simulink model "ClampledRollPID"  (R2025b)
settings: Solver=VariableStepAuto  StartTime=0.0  StopTime=10  RelTol=1e-3
model workspace (MAT data in the model file):
  Dmass = 0.25
  Ix = 0.01
  Iy = 0.01
  Iz = 0.022
  Kd_h = 0
  Kd_r = 5
  Kd_y = 0
  Ki_h = 0
  Ki_r = 1
  Ki_y = 0
  Kp_h = 1
  Kp_r = 4
  Kp_y = 1
  d_m = 1
  d_pitch = 1
  d_roll = 1
  d_yaw = 1
libraries: simulink_extras x1
settings Model: Creator=mariea  LastModifiedBy=mariea
settings SolverCC: ZeroCrossAlgorithm=Adaptive
settings DebuggingCC: IgnoredZcDiagnostic=none

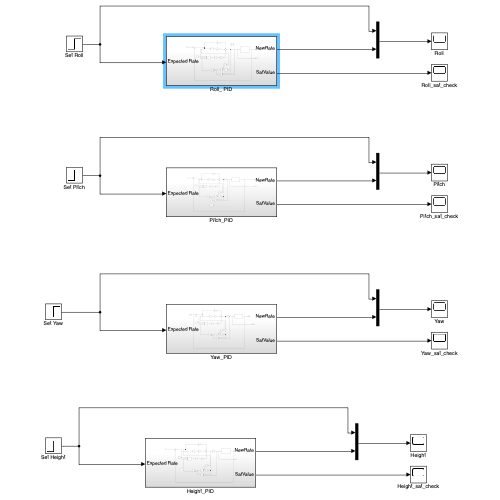
[thumbnail: Simulink's stored preview of the top-level diagram]
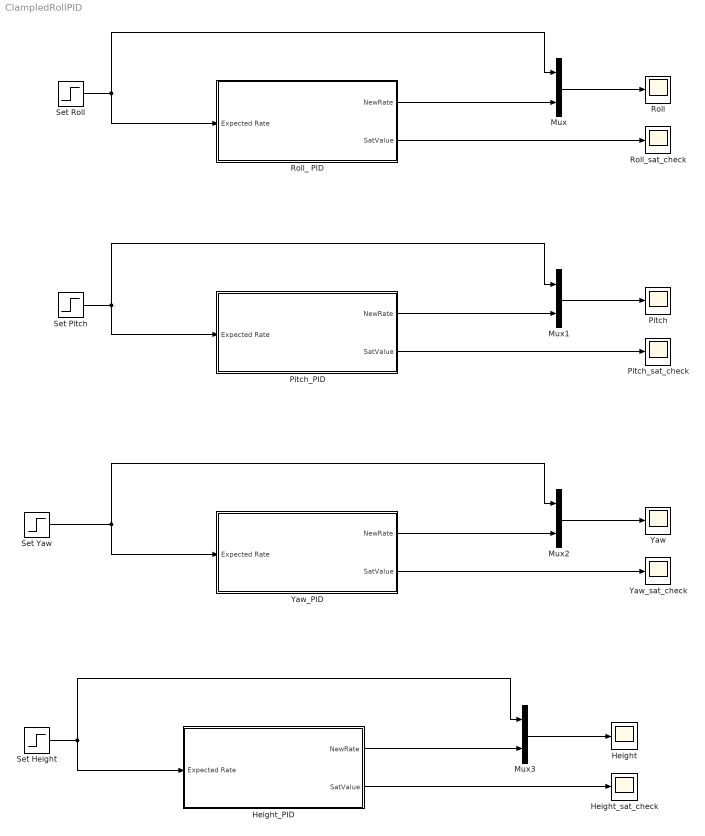
== system ClampledRollPID ==
  Height : Scope
      settings: ActiveDisplayYMinimum=-0.60536887029310371  ActiveDisplayYMaximum=10.192601111350347  DataLoggingVariableName=ScopeData6
  Height_PID : Subsystem
  Height_sat_check : Scope
      settings: ActiveDisplayYMinimum=2.8893405946008759  ActiveDisplayYMaximum=23.442208925875939  DataLoggingVariableName=ScopeData7
  Mux{,1..3} (4 alike) : Mux  Inputs=2
  Pitch : Scope
      settings: ActiveDisplayYMinimum=-0.60536887029310371  ActiveDisplayYMaximum=10.192601111350347  DataLoggingVariableName=ScopeData2
  Pitch_PID : Subsystem
  Pitch_sat_check : Scope
      settings: ActiveDisplayYMinimum=2.8893405946008759  ActiveDisplayYMaximum=23.442208925875939  DataLoggingVariableName=ScopeData3
  Roll : Scope
      settings: ActiveDisplayYMinimum=4.5448731516349712  ActiveDisplayYMaximum=5.1235702214097891
  Roll_ PID : Subsystem
  Roll_sat_check : Scope
      settings: ActiveDisplayYMinimum=-77.252153315942437  ActiveDisplayYMaximum=63.048289708603093
  Set Height : Step  After=3  SampleTime=0
  Set Pitch : Step  After=5  SampleTime=0
  Set Roll : Step  After=10  SampleTime=0
  Set Yaw : Step  After=7  SampleTime=0
  Yaw : Scope
      settings: ActiveDisplayYMinimum=-1.8749999999999996  ActiveDisplayYMaximum=16.875  DataLoggingVariableName=ScopeData4
  Yaw_PID : Subsystem
  Yaw_sat_check : Scope
      settings: ActiveDisplayYMinimum=2.8893405946008759  ActiveDisplayYMaximum=23.442208925875939  DataLoggingVariableName=ScopeData5
  wires:
  Set Roll/1 -> Roll_ PID/1(Expected Rate), Mux/1
  Mux/1 -> Roll/1
  Roll_ PID/1(NewRate) -> Mux/2
  Roll_ PID/2(SatValue) -> Roll_sat_check/1
  Set Pitch/1 -> Pitch_PID/1(Expected Rate), Mux1/1
  Pitch_PID/1(NewRate) -> Mux1/2
  Pitch_PID/2(SatValue) -> Pitch_sat_check/1
  Mux1/1 -> Pitch/1
  Mux2/1 -> Yaw/1
  Yaw_PID/1(NewRate) -> Mux2/2
  Set Yaw/1 -> Yaw_PID/1(Expected Rate), Mux2/1
  Yaw_PID/2(SatValue) -> Yaw_sat_check/1
  Mux3/1 -> Height/1
  Height_PID/1(NewRate) -> Mux3/2
  Set Height/1 -> Height_PID/1(Expected Rate), Mux3/1
  Height_PID/2(SatValue) -> Height_sat_check/1

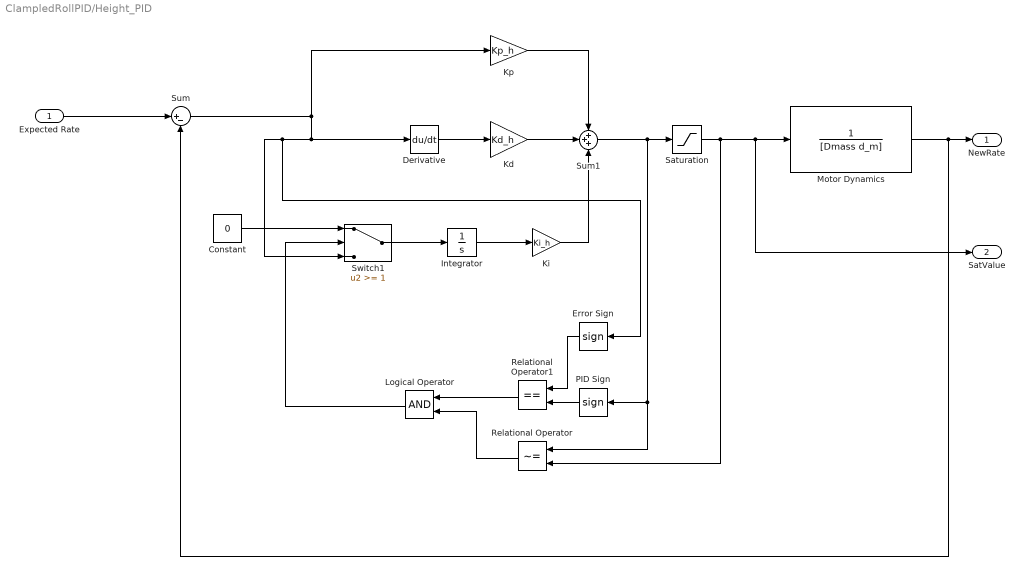
== system ClampledRollPID/Height_PID ==
  Expected Rate : Inport
  Constant : Constant  Value=0
  Derivative : Derivative
  Error Sign : Signum
  Integrator : Integrator
  Kd : Gain  Gain=Kd_h
  Ki : Gain  Gain=Ki_h
  Kp : Gain  Gain=Kp_h
  Logical Operator : Logic  AllPortsSameDT=off  OutDataTypeStr=boolean
  Motor Dynamics : TransferFcn  Denominator=[Dmass d_m]
  PID Sign : Signum
  Relational Operator : RelationalOperator  Operator=~=  OutDataTypeStr=boolean  RndMeth=Simplest  InputSameDT=off
  Relational Operator1 : RelationalOperator  Operator===  OutDataTypeStr=boolean  RndMeth=Simplest  InputSameDT=off
  Saturation : Saturate  UpperLimit=100  LowerLimit=0
  Sum : Sum  Inputs=|+-
  Sum1 : Sum  Inputs=+++
  Switch1 : Switch  Threshold=1  SaturateOnIntegerOverflow=off  InputSameDT=off
  NewRate : Outport
  SatValue : Outport  Port=2
  wires:
  Logical Operator/1 -> Switch1/2
  Kp/1 -> Sum1/1
  Error Sign/1 -> Relational Operator1/1
  Integrator/1 -> Ki/1
  Sum/1 -> Error Sign/1, Switch1/3, Derivative/1, Kp/1
  Switch1/1 -> Integrator/1
  Expected Rate/1 -> Sum/1
  Kd/1 -> Sum1/2
  Ki/1 -> Sum1/3
  Derivative/1 -> Kd/1
  Constant/1 -> Switch1/1
  Relational Operator1/1 -> Logical Operator/1
  Sum1/1 -> Saturation/1, PID Sign/1, Relational Operator/1
  PID Sign/1 -> Relational Operator1/2
  Relational Operator/1 -> Logical Operator/2
  Saturation/1 -> Relational Operator/2, SatValue/1, Motor Dynamics/1
  Motor Dynamics/1 -> Sum/2, NewRate/1

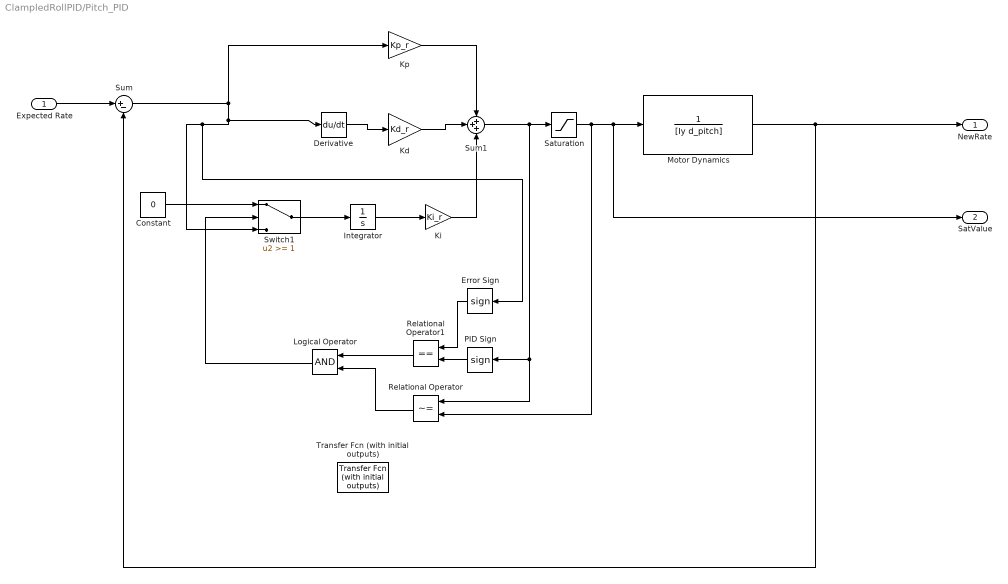
== system ClampledRollPID/Pitch_PID ==
  Expected Rate : Inport
  Constant : Constant  Value=0
  Derivative : Derivative
  Error Sign : Signum
  Integrator : Integrator
  Kd : Gain  Gain=Kd_r
  Ki : Gain  Gain=Ki_r
  Kp : Gain  Gain=Kp_r
  Logical Operator : Logic  AllPortsSameDT=off  OutDataTypeStr=boolean
  Motor Dynamics : TransferFcn  Denominator=[Iy d_pitch]
  PID Sign : Signum
  Relational Operator : RelationalOperator  Operator=~=  OutDataTypeStr=boolean  RndMeth=Simplest  InputSameDT=off
  Relational Operator1 : RelationalOperator  Operator===  OutDataTypeStr=boolean  RndMeth=Simplest  InputSameDT=off
  Saturation : Saturate  UpperLimit=96  LowerLimit=-96
  Sum : Sum  Inputs=|+-
  Sum1 : Sum  Inputs=+++
  Switch1 : Switch  Threshold=1  SaturateOnIntegerOverflow=off  InputSameDT=off
  Transfer Fcn (with initial outputs) : simulink_extras/Additional Linear/Transfer Fcn (with initial outputs)  N=[1]  D="[1  1]"  Y0=.5  U0=0
  NewRate : Outport
  SatValue : Outport  Port=2
  wires:
  Logical Operator/1 -> Switch1/2
  Kp/1 -> Sum1/1
  Error Sign/1 -> Relational Operator1/1
  Integrator/1 -> Ki/1
  Sum/1 -> Error Sign/1, Switch1/3, Derivative/1, Kp/1
  Switch1/1 -> Integrator/1
  Expected Rate/1 -> Sum/1
  Kd/1 -> Sum1/2
  Ki/1 -> Sum1/3
  Derivative/1 -> Kd/1
  Constant/1 -> Switch1/1
  Relational Operator1/1 -> Logical Operator/1
  Sum1/1 -> Saturation/1, PID Sign/1, Relational Operator/1
  Motor Dynamics/1 -> Sum/2, NewRate/1
  PID Sign/1 -> Relational Operator1/2
  Relational Operator/1 -> Logical Operator/2
  Saturation/1 -> SatValue/1, Motor Dynamics/1, Relational Operator/2

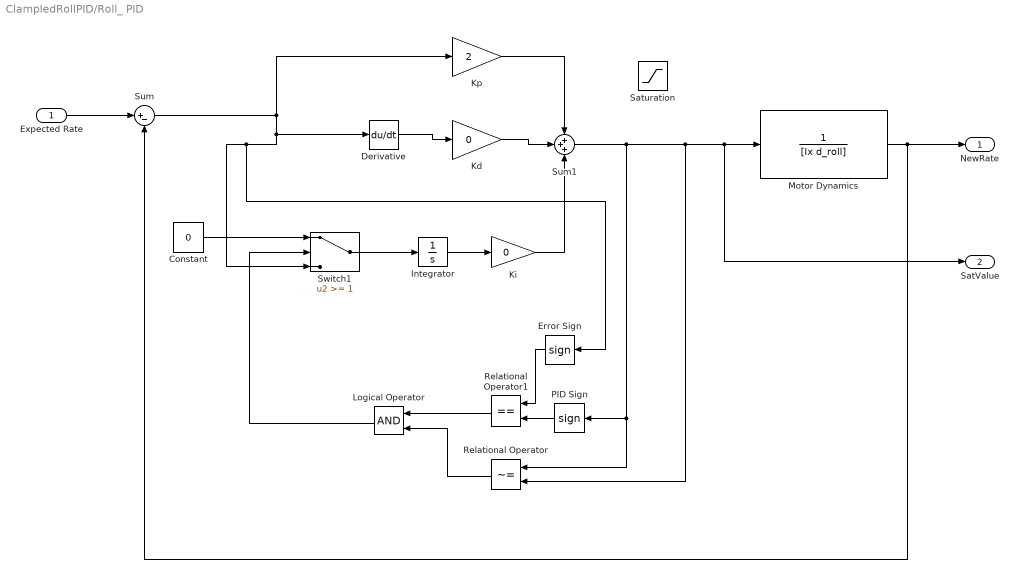
== system ClampledRollPID/Roll_ PID ==
  Expected Rate : Inport
  Constant : Constant  Value=0
  Derivative : Derivative
  Error Sign : Signum
  Integrator : Integrator
  Kd : Gain  Gain=0
  Ki : Gain  Gain=0
  Kp : Gain  Gain=2
  Logical Operator : Logic  AllPortsSameDT=off  OutDataTypeStr=boolean
  Motor Dynamics : TransferFcn  Denominator=[Ix d_roll]
  PID Sign : Signum
  Relational Operator : RelationalOperator  Operator=~=  OutDataTypeStr=boolean  RndMeth=Simplest  InputSameDT=off
  Relational Operator1 : RelationalOperator  Operator===  OutDataTypeStr=boolean  RndMeth=Simplest  InputSameDT=off
  Saturation : Saturate  UpperLimit=96  LowerLimit=-96
  Sum : Sum  Inputs=|+-
  Sum1 : Sum  Inputs=+++
  Switch1 : Switch  Threshold=1  SaturateOnIntegerOverflow=off  InputSameDT=off
  NewRate : Outport
  SatValue : Outport  Port=2
  wires:
  Logical Operator/1 -> Switch1/2
  Kp/1 -> Sum1/1
  Error Sign/1 -> Relational Operator1/1
  Integrator/1 -> Ki/1
  Sum/1 -> Error Sign/1, Switch1/3, Derivative/1, Kp/1
  Switch1/1 -> Integrator/1
  Expected Rate/1 -> Sum/1
  Kd/1 -> Sum1/2
  Ki/1 -> Sum1/3
  Derivative/1 -> Kd/1
  Constant/1 -> Switch1/1
  Relational Operator1/1 -> Logical Operator/1
  Motor Dynamics/1 -> NewRate/1, Sum/2
  PID Sign/1 -> Relational Operator1/2
  Relational Operator/1 -> Logical Operator/2
  Sum1/1 -> SatValue/1, Motor Dynamics/1, Relational Operator/2, PID Sign/1, Relational Operator/1

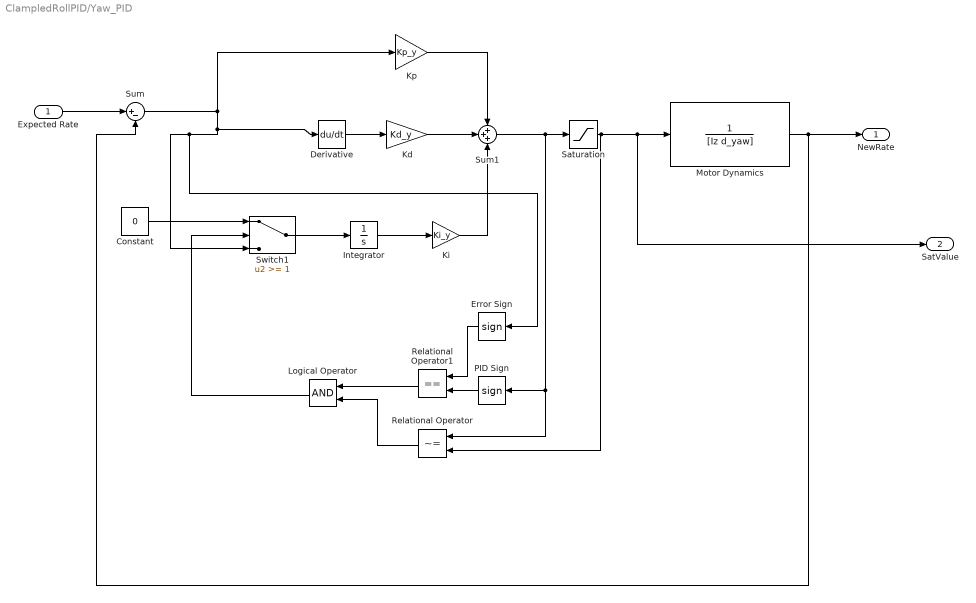
== system ClampledRollPID/Yaw_PID ==
  Expected Rate : Inport
  Constant : Constant  Value=0
  Derivative : Derivative
  Error Sign : Signum
  Integrator : Integrator
  Kd : Gain  Gain=Kd_y
  Ki : Gain  Gain=Ki_y
  Kp : Gain  Gain=Kp_y
  Logical Operator : Logic  AllPortsSameDT=off  OutDataTypeStr=boolean
  Motor Dynamics : TransferFcn  Denominator=[Iz d_yaw]
  PID Sign : Signum
  Relational Operator : RelationalOperator  Operator=~=  OutDataTypeStr=boolean  RndMeth=Simplest  InputSameDT=off
  Relational Operator1 : RelationalOperator  Operator===  OutDataTypeStr=boolean  RndMeth=Simplest  InputSameDT=off
  Saturation : Saturate  UpperLimit=100  LowerLimit=-100
  Sum : Sum  Inputs=|+-
  Sum1 : Sum  Inputs=+++
  Switch1 : Switch  Threshold=1  SaturateOnIntegerOverflow=off  InputSameDT=off
  NewRate : Outport
  SatValue : Outport  Port=2
  wires:
  Logical Operator/1 -> Switch1/2
  Kp/1 -> Sum1/1
  Error Sign/1 -> Relational Operator1/1
  Integrator/1 -> Ki/1
  Sum/1 -> Error Sign/1, Switch1/3, Derivative/1, Kp/1
  Switch1/1 -> Integrator/1
  Expected Rate/1 -> Sum/1
  Kd/1 -> Sum1/2
  Ki/1 -> Sum1/3
  Derivative/1 -> Kd/1
  Constant/1 -> Switch1/1
  Relational Operator1/1 -> Logical Operator/1
  Sum1/1 -> Saturation/1, PID Sign/1, Relational Operator/1
  Motor Dynamics/1 -> NewRate/1, Sum/2
  PID Sign/1 -> Relational Operator1/2
  Relational Operator/1 -> Logical Operator/2
  Saturation/1 -> SatValue/1, Motor Dynamics/1, Relational Operator/2
